simulink subsystem "SimpleStateObserver"  (R2024b)
settings: Solver=VariableStepAuto  StartTime=0.0  StopTime=10.0  RelTol=1e-3
values from neighbouring files (symbols this model uses):
  HwzDen = Hwz.Denominator{1}    [Plant_balrob_calculations.m]
  HwzNum = Hwz.Numerator{1}    [Plant_balrob_calculations.m]
undefined symbols (not defined in the file or in its folder): gbox, sens
settings Model: Creator=federico  LastModifiedBy=Buton

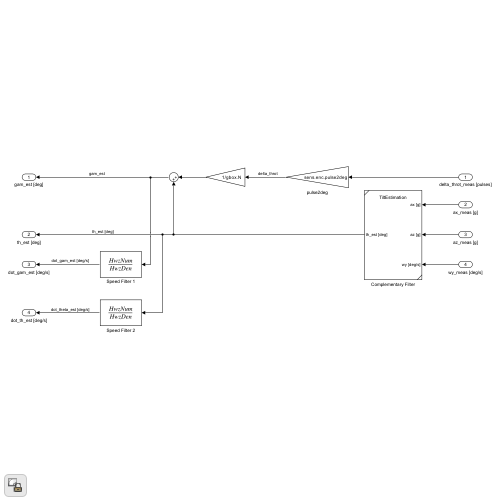
[thumbnail: Simulink's stored preview of the top-level diagram]
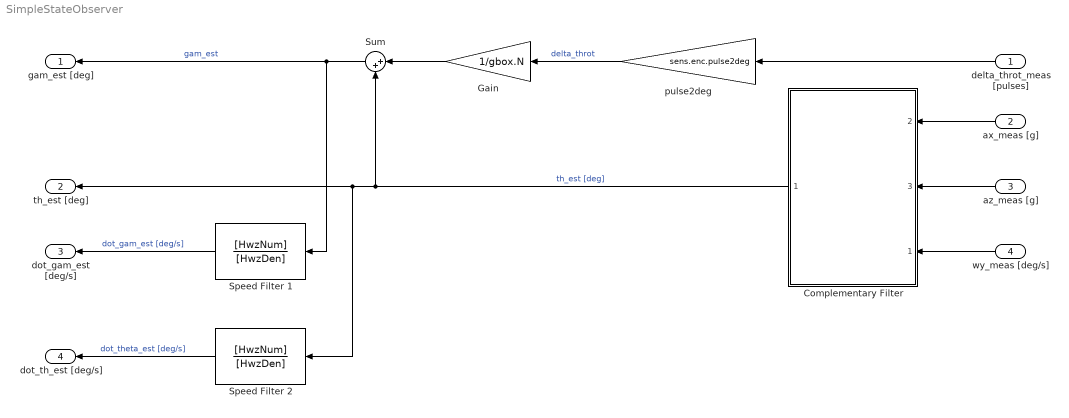
== system SimpleStateObserver ==
  delta_throt_meas [pulses] : Inport
  ax_meas [g] : Inport  Port=2
  az_meas [g] : Inport  Port=3
  wy_meas [deg/s] : Inport  Port=4
  Complementary Filter : Subsystem  ReferencedSubsystem=TiltEstimation
      settings: PortSchema="{\"entries\":[{\"content\":{\"sides\":[{\"content\":{\"connectorIds\":[\"In2\",\"In3\",\"In1\"]},\"type\":\"ConnectorPlacement.EquallySpacedRectSide\",\"uuid\":\"bc9cdf7b-6562-45b3-8ce4-9e9e64b4f4e2\"},{\"content\":{\"connectorIds\":[\"Out1\"],\"side\":\"RIGHT\"},\"type\":\"ConnectorPlacement.EquallySpacedRectSide\",\"uuid\":\"cf9eb48d-95a1-4e60-b0fc-76acb5613ccf\"},{\"content\":{\"side\":\"TOP\"},\"type\":\"ConnectorPlacement.EquallySpacedRectSide\",\"uuid\":\"802ac95a-df21-4b3b-9e69-36b54a9d572d\"}]},\"type\":\"ConnectorPlacement.EquallySpacedConnector\",\"uuid\":\"e2d0de03-3055-44d8-bbda-063517f3a109\"}],\"packageUris\":[\"http://schema.mathworks.com/mf0/Connector/R2020b\"],\"version\":\"1.0\"}"
  Gain : Gain  Gain=1/gbox.N
  Speed Filter 1 : DiscreteTransferFcn  Numerator=[HwzNum]  Denominator=[HwzDen]
  Speed Filter 2 : DiscreteTransferFcn  Numerator=[HwzNum]  Denominator=[HwzDen]
  Sum : Sum  Inputs=|++
  pulse2deg : Gain  Gain=sens.enc.pulse2deg
  gam_est [deg] : Outport
  th_est [deg] : Outport  Port=2
  dot_gam_est [deg/s] : Outport  Port=3
  dot_th_est [deg/s] : Outport  Port=4
  wires:
  ax_meas [g]/1 -> Complementary Filter/2
  az_meas [g]/1 -> Complementary Filter/3
  wy_meas [deg/s]/1 -> Complementary Filter/1
  delta_throt_meas [pulses]/1 -> pulse2deg/1
  pulse2deg/1 -> Gain/1  "delta_throt"
  Gain/1 -> Sum/1
  Complementary Filter/1 -> Speed Filter 2/1, th_est [deg]/1, Sum/2  "th_est [deg]"
  Sum/1 -> gam_est [deg]/1, Speed Filter 1/1  "gam_est"
  Speed Filter 1/1 -> dot_gam_est [deg/s]/1  "dot_gam_est [deg/s]"
  Speed Filter 2/1 -> dot_th_est [deg/s]/1  "dot_theta_est [deg/s]"
